simulink model "pg7"  (R2025a)
settings: Solver=VariableStepAuto  StartTime=0.0  StopTime=100  RelTol=1e-3
libraries: dspfdesign x2
settings Model: Creator=Student  LastModifiedBy=Student

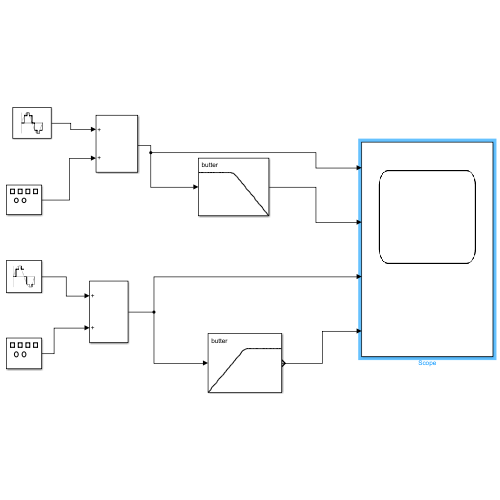
[thumbnail: Simulink's stored preview of the top-level diagram]
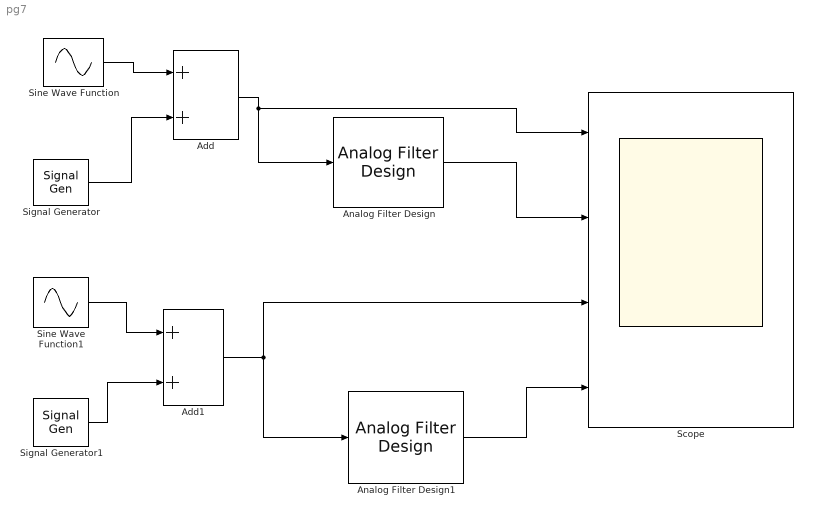
== system pg7 ==
  Add : Sum
  Add1 : Sum
  Analog Filter Design : dspfdesign/Analog Filter Design  method=Butterworth  filttype=Lowpass  N=8  Wlo=30  Whi=80  Rp=2  Rs=40
  Analog Filter Design1 : dspfdesign/Analog Filter Design  method=Butterworth  filttype=Highpass  N=8  Wlo=10  Whi=80  Rp=2  Rs=40
  Scope : Scope  NumInputPorts=4
      settings: ActiveDisplayString=4  ActiveDisplayYMinimum=-6.2179598478864371  ActiveDisplayYMaximum=6.2408301561321959
  Signal Generator : SignalGenerator  WaveForm=random  Amplitude=2  Frequency=200  Units=rad/sec
  Signal Generator1 : SignalGenerator  WaveForm=random  Frequency=100  Units=rad/sec
  Sine Wave Function : Sin  Amplitude=3  Frequency=50  SampleTime=1
  Sine Wave Function1 : Sin  Amplitude=3  Frequency=200  SampleTime=1
  wires:
  Sine Wave Function/1 -> Add/1
  Signal Generator/1 -> Add/2
  Sine Wave Function1/1 -> Add1/1
  Signal Generator1/1 -> Add1/2
  Add1/1 -> Scope/3, Analog Filter Design1/1
  Add/1 -> Scope/1, Analog Filter Design/1
  Analog Filter Design/1 -> Scope/2
  Analog Filter Design1/1 -> Scope/4
